simulink model "SoRo_Compliant_Demo_0906"  (R2023b)
settings: Solver=FixedStepAuto  StartTime=0.0  StopTime=inf  FixedStep=0.01  RelTol=1e-3
undefined symbols (not defined in the file): Down, Pull
libraries: simulink x50, speedgoatlib_IO691 x20, canmsglib x19, slpidlib x12, dspfdesign x6
(part 3 of 3)

== system SoRo_Compliant_Demo_0906/Tension_Mode_flag=2/Subsystem2 ==
  tension_in : Inport
  position_in : Inport  Port=2
  Enable : EnablePort
  tension_out : Outport
  position_out : Outport  Port=2
  wires:
  position_in/1 -> position_out/1
  tension_in/1 -> tension_out/1

== system SoRo_Compliant_Demo_0906/Tension_Mode_flag=2/Subsystem3 ==
  tension_in : Inport
  position_in : Inport  Port=2
  Enable : EnablePort
  tension_out : Outport
  position_out : Outport  Port=2
  wires:
  tension_in/1 -> tension_out/1
  position_in/1 -> position_out/1

== system SoRo_Compliant_Demo_0906/Tension_adjust_flag=4/Subsystem1 ==
  InitialSwitchValue_in : Inport
  Enable : EnablePort
  InitialSwitchValue_out : Outport
  wires:
  InitialSwitchValue_in/1 -> InitialSwitchValue_out/1

== system SoRo_Compliant_Demo_0906/Tension_adjust_flag=4/Subsystem4 ==
  tension_in : Inport
  position_in : Inport  Port=2
  Enable : EnablePort
  tension_out : Outport
  position_out : Outport  Port=2
  wires:
  tension_in/1 -> tension_out/1
  position_in/1 -> position_out/1

== system SoRo_Compliant_Demo_0906/Tension_adjust_flag=4/Subsystem5 ==
  tension_in : Inport
  position_in : Inport  Port=2
  Enable : EnablePort
  tension_out : Outport
  position_out : Outport  Port=2
  wires:
  tension_in/1 -> tension_out/1
  position_in/1 -> position_out/1

== system SoRo_Compliant_Demo_0906/Tension_adjust_flag=4/Subsystem6 ==
  tension_in : Inport
  position_in : Inport  Port=2
  Enable : EnablePort
  tension_out : Outport
  position_out : Outport  Port=2
  wires:
  position_in/1 -> position_out/1
  tension_in/1 -> tension_out/1

== system SoRo_Compliant_Demo_0906/Tension_adjust_flag=4/Subsystem7 ==
  tension_in : Inport
  position_in : Inport  Port=2
  Enable : EnablePort
  tension_out : Outport
  position_out : Outport  Port=2
  wires:
  tension_in/1 -> tension_out/1
  position_in/1 -> position_out/1

== system SoRo_Compliant_Demo_0906/Transmit/Driver_Upload ==
  Enable : EnablePort  StatesWhenEnabling=reset
  CAN Pack : canmsglib/CAN Pack  CANdbFile=E:\OneDrive\OneDrive - The Chinese University of Hong Kong\文档\Research\SRIL\12nd\Experiment\Simulink\RoboModule0729.dbc  MsgList=Configuration_all  MsgName=Configuration_all  MsgIDType=Standard (11-bit identifier)  MsgIdentifier=10  MsgLength=8  Remote=off  ApplyMinMax=off  BusOutput=off  SignalInfo={'Data2','16','8','BE','unsigned','Standard','0','1','0','-Inf','Inf';'Data3','24','8','BE','unsigned','Standard','0','1','0','-Inf','Inf';'Data4','32','8','BE','unsigned','Standard','0','1','0','-Inf','Inf';'Data5','40','8','BE','unsigned','Standard','0','1','0','-Inf','Inf';'Data6','48','8','BE','unsigned','Standard','0','1','0','-Inf','Inf';'Data7','56','8','BE','unsigned','Standard','0','1','0','-Inf','Inf';'output_cycle_curvelpos','0','8','BE','unsigned','Standard','0','1','0','-Inf','Inf';'output_cycle_others','8','8','BE','unsigned','Standard','0','1','0','-Inf','Inf'}
      settings: DataFormat=CANdb specified signals
  "CAN Write " : speedgoatlib_IO691/CAN Write   moduleType=IO691  id=1  channel=1  canType=CAN (HS)  messageType=CAN (HS)  useBusIn=off  numOfMsg=1  enableInput=off  enableStatusPort=off  ts=-1  initValues=[691 1 -1 0 1 1 0 1 0 0]
      settings: SourceProductName=Simulink Real-Time: Speedgoat I/O Blockset
  Constant4 : Constant  Value=hex2dec('0x55')  OutDataTypeStr=uint8  SampleTime=-1
  Constant5 : Constant  Value=hex2dec('0x64')  OutDataTypeStr=uint8  SampleTime=-1
  Constant6 : Constant  Value=hex2dec('0x00')  OutDataTypeStr=uint8  SampleTime=-1
  wires:
  CAN Pack/1 -> "CAN Write "/1
  Constant4/1 -> CAN Pack/1, CAN Pack/3, CAN Pack/5, CAN Pack/6, CAN Pack/4, CAN Pack/2
  Constant5/1 -> CAN Pack/7
  Constant6/1 -> CAN Pack/8

== system SoRo_Compliant_Demo_0906/Transmit/Mode Selection ==
  Enable : EnablePort  StatesWhenEnabling=reset
  CAN Pack : canmsglib/CAN Pack  CANdbFile=E:\Research\SRIL\12nd\Simulink\RoboModule0729.dbc  MsgList=Mode_Selection_all  MsgName=Mode_Selection_all  MsgIDType=Standard (11-bit identifier)  MsgIdentifier=1  MsgLength=8  Remote=off  ApplyMinMax=off  BusOutput=off  SignalInfo={'Data1','8','8','BE','unsigned','Standard','0','1','0','-Inf','Inf';'Data2','16','8','BE','unsigned','Standard','0','1','0','-Inf','Inf';'Data3','24','8','BE','unsigned','Standard','0','1','0','-Inf','Inf';'Data4','32','8','BE','unsigned','Standard','0','1','0','-Inf','Inf';'Data5','40','8','BE','unsigned','Standard','0','1','0','-Inf','Inf';'Data6','48','8','BE','unsigned','Standard','0','1','0','-Inf','Inf';'Data7','56','8','BE','unsigned','Standard','0','1','0','-Inf','Inf';'Mode','0','8','BE','unsigned','Standard','0','1','0','-Inf','Inf'}
      settings: DataFormat=CANdb specified signals
  "CAN Write " : speedgoatlib_IO691/CAN Write   moduleType=IO691  id=1  channel=1  canType=CAN (HS)  messageType=CAN (HS)  useBusIn=off  numOfMsg=1  enableInput=off  enableStatusPort=off  ts=-1  initValues=[691 1 -1 0 1 1 0 1 0 0]
      settings: SourceProductName=Simulink Real-Time: Speedgoat I/O Blockset
  Constant2 : Constant  Value=hex2dec('0x55')  OutDataTypeStr=uint8  SampleTime=-1
  Mode Number1 : Constant  Value=hex2dec('0x04')  OutDataTypeStr=uint8  SampleTime=-1
  wires:
  Constant2/1 -> CAN Pack/1, CAN Pack/3, CAN Pack/5, CAN Pack/6, CAN Pack/7, CAN Pack/4, CAN Pack/2
  CAN Pack/1 -> "CAN Write "/1
  Mode Number1/1 -> CAN Pack/8

== system SoRo_Compliant_Demo_0906/Transmit/PosSpdMode1 ==
  note: R ated Voltage of Motor is 12 V. Supply Voltage is 24 V. Limilation of the temp_pwm is set as 2500.
  Inport2 : Inport
  Enable : EnablePort
  CAN Pack : canmsglib/CAN Pack  CANdbFile=E:\OneDrive\OneDrive - The Chinese University of Hong Kong\文档\Research\SRIL\12nd\Experiment\Simulink\RoboModule0729.dbc  MsgList=Position_Dr1  MsgName=Position_Dr1  MsgIDType=Standard (11-bit identifier)  MsgIdentifier=21  MsgLength=8  Remote=off  ApplyMinMax=off  BusOutput=off  SignalInfo={'Data2','16','8','BE','unsigned','Standard','0','1','0','-Inf','Inf';'Data3','24','8','BE','unsigned','Standard','0','1','0','-Inf','Inf';'temp_position','56','32','BE','signed','Standard','0','1','0','-Inf','Inf';'temp_pwm','8','16','BE','unsigned','Standard','0','1','0','-Inf','Inf'}
      settings: DataFormat=CANdb specified signals
  "CAN Write " : speedgoatlib_IO691/CAN Write   moduleType=IO691  id=1  channel=1  canType=CAN (HS)  messageType=CAN (HS)  useBusIn=off  numOfMsg=1  enableInput=off  enableStatusPort=off  ts=-1  initValues=[691 1 -1 0 1 1 0 1 0 0]
      settings: SourceProductName=Simulink Real-Time: Speedgoat I/O Blockset
  Constant1 : Constant  Value=5000
  Constant3 : Constant  Value=hex2dec('0x55')  OutDataTypeStr=uint8  SampleTime=-1
  wires:
  Constant3/1 -> CAN Pack/2, CAN Pack/1
  Inport2/1 -> CAN Pack/3
  Constant1/1 -> CAN Pack/4
  CAN Pack/1 -> "CAN Write "/1

== system SoRo_Compliant_Demo_0906/Transmit/PosSpdMode2 ==
  note: R ated Voltage of Motor is 12 V. Supply Voltage is 24 V. Limilation of the temp_pwm is set as 2500.
  Inport2 : Inport
  Enable : EnablePort
  CAN Pack : canmsglib/CAN Pack  CANdbFile=E:\Research\SRIL\12nd\Simulink\RoboModule0729.dbc  MsgList=Position_Dr2  MsgName=Position_Dr2  MsgIDType=Standard (11-bit identifier)  MsgIdentifier=37  MsgLength=8  Remote=off  ApplyMinMax=off  BusOutput=off  SignalInfo={'Data2','16','8','BE','unsigned','Standard','0','1','0','-Inf','Inf';'Data3','24','8','BE','unsigned','Standard','0','1','0','-Inf','Inf';'temp_position','56','32','BE','signed','Standard','0','1','0','-Inf','Inf';'temp_pwm','8','16','BE','unsigned','Standard','0','1','0','-Inf','Inf'}
      settings: DataFormat=CANdb specified signals
  "CAN Write " : speedgoatlib_IO691/CAN Write   moduleType=IO691  id=1  channel=1  canType=CAN (HS)  messageType=CAN (HS)  useBusIn=off  numOfMsg=1  enableInput=off  enableStatusPort=off  ts=-1  initValues=[691 1 -1 0 1 1 0 1 0 0]
      settings: SourceProductName=Simulink Real-Time: Speedgoat I/O Blockset
  Constant1 : Constant  Value=5000
  Constant3 : Constant  Value=hex2dec('0x55')  OutDataTypeStr=uint8  SampleTime=-1
  Scope : Scope
  wires:
  CAN Pack/1 -> "CAN Write "/1
  Constant3/1 -> CAN Pack/2, CAN Pack/1
  Inport2/1 -> Scope/1, CAN Pack/3
  Constant1/1 -> CAN Pack/4

== system SoRo_Compliant_Demo_0906/Transmit/PosSpdMode3 ==
  note: R ated Voltage of Motor is 12 V. Supply Voltage is 24 V. Limilation of the temp_pwm is set as 2500.
  Inport2 : Inport
  Enable : EnablePort
  CAN Pack : canmsglib/CAN Pack  CANdbFile=E:\OneDrive\OneDrive - The Chinese University of Hong Kong\文档\Research\SRIL\12nd\Experiment\Simulink\RoboModule0729.dbc  MsgList=Position_Dr3  MsgName=Position_Dr3  MsgIDType=Standard (11-bit identifier)  MsgIdentifier=53  MsgLength=8  Remote=off  ApplyMinMax=off  BusOutput=off  SignalInfo={'Data2','16','8','BE','unsigned','Standard','0','1','0','-Inf','Inf';'Data3','24','8','BE','unsigned','Standard','0','1','0','-Inf','Inf';'temp_position','56','32','BE','signed','Standard','0','1','0','-Inf','Inf';'temp_pwm','8','16','BE','unsigned','Standard','0','1','0','-Inf','Inf'}
      settings: DataFormat=CANdb specified signals
  "CAN Write " : speedgoatlib_IO691/CAN Write   moduleType=IO691  id=1  channel=1  canType=CAN (HS)  messageType=CAN (HS)  useBusIn=off  numOfMsg=1  enableInput=off  enableStatusPort=off  ts=-1  initValues=[691 1 -1 0 1 1 0 1 0 0]
      settings: SourceProductName=Simulink Real-Time: Speedgoat I/O Blockset
  Constant1 : Constant  Value=5000
  Constant3 : Constant  Value=hex2dec('0x55')  OutDataTypeStr=uint8  SampleTime=-1
  wires:
  CAN Pack/1 -> "CAN Write "/1
  Constant3/1 -> CAN Pack/2, CAN Pack/1
  Inport2/1 -> CAN Pack/3
  Constant1/1 -> CAN Pack/4

== system SoRo_Compliant_Demo_0906/Transmit/PosSpdMode4 ==
  note: R ated Voltage of Motor is 12 V. Supply Voltage is 24 V. Limilation of the temp_pwm is set as 2500.
  Inport2 : Inport
  Enable : EnablePort
  CAN Pack : canmsglib/CAN Pack  CANdbFile=E:\OneDrive\OneDrive - The Chinese University of Hong Kong\文档\Research\SRIL\12nd\Experiment\Simulink\RoboModule0729.dbc  MsgList=Position_Dr4  MsgName=Position_Dr4  MsgIDType=Standard (11-bit identifier)  MsgIdentifier=69  MsgLength=8  Remote=off  ApplyMinMax=off  BusOutput=off  SignalInfo={'Data2','16','8','BE','unsigned','Standard','0','1','0','-Inf','Inf';'Data3','24','8','BE','unsigned','Standard','0','1','0','-Inf','Inf';'temp_position','56','32','BE','signed','Standard','0','1','0','-Inf','Inf';'temp_pwm','8','16','BE','unsigned','Standard','0','1','0','-Inf','Inf'}
      settings: DataFormat=CANdb specified signals
  "CAN Write " : speedgoatlib_IO691/CAN Write   moduleType=IO691  id=1  channel=1  canType=CAN (HS)  messageType=CAN (HS)  useBusIn=off  numOfMsg=1  enableInput=off  enableStatusPort=off  ts=-1  initValues=[691 1 -1 0 1 1 0 1 0 0]
      settings: SourceProductName=Simulink Real-Time: Speedgoat I/O Blockset
  Constant1 : Constant  Value=5000
  Constant3 : Constant  Value=hex2dec('0x55')  OutDataTypeStr=uint8  SampleTime=-1
  wires:
  CAN Pack/1 -> "CAN Write "/1
  Constant3/1 -> CAN Pack/2, CAN Pack/1
  Inport2/1 -> CAN Pack/3
  Constant1/1 -> CAN Pack/4

== system SoRo_Compliant_Demo_0906/Transmit/PosSpdMode5 ==
  note: R ated Voltage of Motor is 12 V. Supply Voltage is 24 V. Limilation of the temp_pwm is set as 2500.
  Inport2 : Inport
  Enable : EnablePort
  CAN Pack : canmsglib/CAN Pack  CANdbFile=E:\OneDrive\OneDrive - The Chinese University of Hong Kong\文档\Research\SRIL\12nd\Experiment\Simulink\RoboModule0729.dbc  MsgList=Position_Dr5  MsgName=Position_Dr5  MsgIDType=Standard (11-bit identifier)  MsgIdentifier=85  MsgLength=8  Remote=off  ApplyMinMax=off  BusOutput=off  SignalInfo={'Data2','16','8','BE','unsigned','Standard','0','1','0','-Inf','Inf';'Data3','24','8','BE','unsigned','Standard','0','1','0','-Inf','Inf';'temp_position','56','32','BE','signed','Standard','0','1','0','-Inf','Inf';'temp_pwm','8','16','BE','unsigned','Standard','0','1','0','-Inf','Inf'}
      settings: DataFormat=CANdb specified signals
  "CAN Write " : speedgoatlib_IO691/CAN Write   moduleType=IO691  id=1  channel=1  canType=CAN (HS)  messageType=CAN (HS)  useBusIn=off  numOfMsg=1  enableInput=off  enableStatusPort=off  ts=-1  initValues=[691 1 -1 0 1 1 0 1 0 0]
      settings: SourceProductName=Simulink Real-Time: Speedgoat I/O Blockset
  Constant1 : Constant  Value=5000
  Constant3 : Constant  Value=hex2dec('0x55')  OutDataTypeStr=uint8  SampleTime=-1
  Scope : Scope
  wires:
  CAN Pack/1 -> "CAN Write "/1
  Constant3/1 -> CAN Pack/2, CAN Pack/1
  Inport2/1 -> Scope/1, CAN Pack/3
  Constant1/1 -> CAN Pack/4

== system SoRo_Compliant_Demo_0906/Transmit/Reset ==
  Enable : EnablePort  StatesWhenEnabling=reset
  CAN Pack : canmsglib/CAN Pack  CANdbFile=E:\Research\SRIL\12nd\Simulink\RoboModule0729.dbc  MsgList=Reset_all  MsgName=Reset_all  MsgIDType=Standard (11-bit identifier)  MsgIdentifier=0  MsgLength=8  Remote=off  ApplyMinMax=off  BusOutput=off  SignalInfo={'Data0','0','8','BE','unsigned','Standard','0','1','0','-Inf','Inf';'Data1','8','8','BE','unsigned','Standard','0','1','0','-Inf','Inf';'Data2','16','8','BE','unsigned','Standard','0','1','0','-Inf','Inf';'Data3','24','8','BE','unsigned','Standard','0','1','0','-Inf','Inf';'Data4','32','8','BE','unsigned','Standard','0','1','0','-Inf','Inf';'Data5','40','8','BE','unsigned','Standard','0','1','0','-Inf','Inf';'Data6','48','8','BE','unsigned','Standard','0','1','0','-Inf','Inf';'Data7','56','8','BE','unsigned','Standard','0','1','0','-Inf','Inf'}
      settings: DataFormat=CANdb specified signals
  "CAN Write " : speedgoatlib_IO691/CAN Write   moduleType=IO691  id=1  channel=1  canType=CAN (HS)  messageType=CAN (HS)  useBusIn=off  numOfMsg=1  enableInput=off  enableStatusPort=off  ts=-1  initValues=[691 1 -1 0 1 1 0 1 0 0]
      settings: SourceProductName=Simulink Real-Time: Speedgoat I/O Blockset
  Constant2 : Constant  Value=hex2dec('0x55')  OutDataTypeStr=uint8  SampleTime=-1
  wires:
  CAN Pack/1 -> "CAN Write "/1
  Constant2/1 -> CAN Pack/1, CAN Pack/3, CAN Pack/5, CAN Pack/6, CAN Pack/7, CAN Pack/8, CAN Pack/4, CAN Pack/2

== system SoRo_Compliant_Demo_0906/Transmit/Reset_Manually ==
  Enable : EnablePort  StatesWhenEnabling=reset
  Trigger : TriggerPort  VariantControl=(inherit)  PortDimensions=1
  CAN Pack : canmsglib/CAN Pack  CANdbFile=E:\OneDrive\OneDrive - The Chinese University of Hong Kong\文档\Research\SRIL\12nd\Experiment\Simulink\RoboModule0729.dbc  MsgList=Reset_all  MsgName=Reset_all  MsgIDType=Standard (11-bit identifier)  MsgIdentifier=0  MsgLength=8  Remote=off  ApplyMinMax=off  BusOutput=off  SignalInfo={'Data0','0','8','BE','unsigned','Standard','0','1','0','-Inf','Inf';'Data1','8','8','BE','unsigned','Standard','0','1','0','-Inf','Inf';'Data2','16','8','BE','unsigned','Standard','0','1','0','-Inf','Inf';'Data3','24','8','BE','unsigned','Standard','0','1','0','-Inf','Inf';'Data4','32','8','BE','unsigned','Standard','0','1','0','-Inf','Inf';'Data5','40','8','BE','unsigned','Standard','0','1','0','-Inf','Inf';'Data6','48','8','BE','unsigned','Standard','0','1','0','-Inf','Inf';'Data7','56','8','BE','unsigned','Standard','0','1','0','-Inf','Inf'}
      settings: DataFormat=CANdb specified signals
  "CAN Write " : speedgoatlib_IO691/CAN Write   moduleType=IO691  id=1  channel=1  canType=CAN (HS)  messageType=CAN (HS)  useBusIn=off  numOfMsg=1  enableInput=off  enableStatusPort=off  ts=-1  initValues=[691 1 -1 0 1 1 0 1 0 0]
      settings: SourceProductName=Simulink Real-Time: Speedgoat I/O Blockset
  Constant2 : Constant  Value=hex2dec('0x55')  OutDataTypeStr=uint8  SampleTime=-1
  wires:
  CAN Pack/1 -> "CAN Write "/1
  Constant2/1 -> CAN Pack/1, CAN Pack/3, CAN Pack/5, CAN Pack/6, CAN Pack/7, CAN Pack/8, CAN Pack/4, CAN Pack/2

== system SoRo_Compliant_Demo_0906/Displacement_mode_flag=5/Displacement_mode_flag=0/Subsystem1 ==
  position_in : Inport
  Enable : EnablePort
  position_out : Outport
  wires:
  position_in/1 -> position_out/1

== system SoRo_Compliant_Demo_0906/Displacement_mode_flag=5/Displacement_mode_flag=0/Subsystem2 ==
  position_in : Inport
  Enable : EnablePort
  position_out : Outport
  wires:
  position_in/1 -> position_out/1

== system SoRo_Compliant_Demo_0906/Displacement_mode_flag=5/Displacement_mode_flag=0/Subsystem3 ==
  position_in : Inport
  Enable : EnablePort
  position_out : Outport
  wires:
  position_in/1 -> position_out/1

== system SoRo_Compliant_Demo_0906/Displacement_mode_flag=5/Displacement_mode_flag=0/Subsystem5 ==
  position_in : Inport
  Enable : EnablePort
  position_out : Outport
  wires:
  position_in/1 -> position_out/1

== system SoRo_Compliant_Demo_0906/Displacement_mode_flag=5/Displacement_mode_flag=1/Subsystem1 ==
  position_in : Inport
  Enable : EnablePort
  position_out : Outport
  wires:
  position_in/1 -> position_out/1

== system SoRo_Compliant_Demo_0906/Displacement_mode_flag=5/Displacement_mode_flag=1/Subsystem2 ==
  position_in : Inport
  Enable : EnablePort
  position_out : Outport
  wires:
  position_in/1 -> position_out/1

== system SoRo_Compliant_Demo_0906/Displacement_mode_flag=5/Displacement_mode_flag=1/Subsystem3 ==
  position_in : Inport
  Enable : EnablePort
  position_out : Outport
  wires:
  position_in/1 -> position_out/1

== system SoRo_Compliant_Demo_0906/Displacement_mode_flag=5/Displacement_mode_flag=1/Subsystem5 ==
  position_in : Inport
  Enable : EnablePort
  position_out : Outport
  wires:
  position_in/1 -> position_out/1

== system SoRo_Compliant_Demo_0906/Displacement_mode_flag=5/Displacement_mode_flag=2/Subsystem1 ==
  position_in : Inport
  Enable : EnablePort
  position_out : Outport
  wires:
  position_in/1 -> position_out/1

== system SoRo_Compliant_Demo_0906/Displacement_mode_flag=5/Displacement_mode_flag=2/Subsystem2 ==
  position_in : Inport
  Enable : EnablePort
  position_out : Outport
  wires:
  position_in/1 -> position_out/1

== system SoRo_Compliant_Demo_0906/Displacement_mode_flag=5/Displacement_mode_flag=2/Subsystem3 ==
  position_in : Inport
  Enable : EnablePort
  position_out : Outport
  wires:
  position_in/1 -> position_out/1

== system SoRo_Compliant_Demo_0906/Displacement_mode_flag=5/Displacement_mode_flag=2/Subsystem5 ==
  position_in : Inport
  Enable : EnablePort
  position_out : Outport
  wires:
  position_in/1 -> position_out/1

== system SoRo_Compliant_Demo_0906/Displacement_mode_flag=5/Displacement_mode_flag=3/Subsystem1 ==
  position_in : Inport
  Enable : EnablePort
  position_out : Outport
  wires:
  position_in/1 -> position_out/1

== system SoRo_Compliant_Demo_0906/Displacement_mode_flag=5/Displacement_mode_flag=3/Subsystem2 ==
  position_in : Inport
  Enable : EnablePort
  position_out : Outport
  wires:
  position_in/1 -> position_out/1

== system SoRo_Compliant_Demo_0906/Displacement_mode_flag=5/Displacement_mode_flag=3/Subsystem3 ==
  position_in : Inport
  Enable : EnablePort
  position_out : Outport
  wires:
  position_in/1 -> position_out/1

== system SoRo_Compliant_Demo_0906/Displacement_mode_flag=5/Displacement_mode_flag=3/Subsystem5 ==
  position_in : Inport
  Enable : EnablePort
  position_out : Outport
  wires:
  position_in/1 -> position_out/1

== system SoRo_Compliant_Demo_0906/Displacement_mode_flag=5/Displacement_mode_flag=4/Subsystem1 ==
  position_in : Inport
  Enable : EnablePort
  position_out : Outport
  wires:
  position_in/1 -> position_out/1

== system SoRo_Compliant_Demo_0906/Displacement_mode_flag=5/Displacement_mode_flag=4/Subsystem2 ==
  position_in : Inport
  Enable : EnablePort
  position_out : Outport
  wires:
  position_in/1 -> position_out/1

== system SoRo_Compliant_Demo_0906/Displacement_mode_flag=5/Displacement_mode_flag=4/Subsystem3 ==
  position_in : Inport
  Enable : EnablePort
  position_out : Outport
  wires:
  position_in/1 -> position_out/1

== system SoRo_Compliant_Demo_0906/Displacement_mode_flag=5/Displacement_mode_flag=4/Subsystem5 ==
  position_in : Inport
  Enable : EnablePort
  position_out : Outport
  wires:
  position_in/1 -> position_out/1

== stateflow chart SoRo_Compliant_Demo_0906/Chart2 ==
  settings: sampleTime=0.001
  note: Operation logic: The initial flag is 0. Imitating the operation logic of the drone, long press the H switch for 5 seconds, the flag changes to 1, and the system starts. Long press again for 5 seconds, and the flag changes back to 0.
  state b [parallel]
    settings: executionOrder=1
    state off
      during:flag=0;
    state Initial
      during:flag=1;
    state Tension_Mode
      during:flag=2;
    state Displacement_Mode
      during:flag=3;
    state Individual_Adjust
      during:flag=5;
    state Stiffness_Adjust
      during:flag=4;
    state Emergency_Brake
      during:flag=6;
    Individual_Adjust -> off [order 3] : [duration(Switch_H > 1000) > 3]
    Displacement_Mode -> off [order 2] : [duration(Switch_H > 1000) > 3]
    Tension_Mode -> off [order 3] : [duration(Switch_H > 1000) > 3]
    Displacement_Mode -> Tension_Mode [order 1] : [Switch_B_Change > 0]
    Displacement_Mode -> Individual_Adjust [order 4] : [Switch_D_Change > 0]
    Initial -> Tension_Mode [order 2] : [Switch_A_Change > 0]
    Initial -> off [order 1] : [duration(Switch_H > 1000) > 3]
    (default) -> off
    Tension_Mode -> Initial [order 1] : [Switch_A_Change > 0]
    Individual_Adjust -> Displacement_Mode [order 1] : [Switch_D_Change > 0]
    off -> Initial : [duration(Switch_H > 1000) > 3]
    Tension_Mode -> Displacement_Mode [order 2] : [Switch_B_Change > 0]
    Initial -> Emergency_Brake [order 3] : [Switch_C_Change > 0]
    Tension_Mode -> Stiffness_Adjust [order 5] : [Switch_E_Change > 0]
    Stiffness_Adjust -> Tension_Mode [order 3] : [Switch_E_Change > 0]
    Tension_Mode -> Emergency_Brake [order 4] : [Switch_C_Change > 0]
    Displacement_Mode -> Emergency_Brake [order 3] : [Switch_C_Change > 0]
    Individual_Adjust -> Emergency_Brake [order 2] : [Switch_C_Change > 0]
    Stiffness_Adjust -> off [order 1] : [duration(Switch_H > 1000) > 3]
    Stiffness_Adjust -> Emergency_Brake [order 2] : [Switch_C_Change > 0]
  data: flag output double; Switch_A_Change input double; Switch_E_Change input double; Switch_H input double; Switch_B_Change input double; Switch_C_Change input double; Switch_D_Change input double

== matlab function SoRo_Compliant_Demo_0906/MATLAB Function4 ==
  data: y output; u_out output; u input; u_last input
function [y,u_out] = fcn(u,u_last)
if abs(u-u_last)>20
    y = 1;
else
    y = 0;
end
u_out = u;

== matlab function SoRo_Compliant_Demo_0906/Tension_Mode_flag=2/MATLAB Function1 ==
  data: y output; u input; threshold input
function y = noise_reduction(u,threshold)
if abs(u - 1000) > threshold
    y = u;
else
    y = 1000;
end

== matlab function SoRo_Compliant_Demo_0906/MATLAB Function1 ==
  data: y output; u_out output; u input; u_last input
function [y,u_out] = fcn(u,u_last)
if abs(u-u_last)>20
    y = 1;
else
    y = 0;
end
u_out = u;

== matlab function SoRo_Compliant_Demo_0906/MATLAB Function2 ==
  data: y output; u_out output; u input; u_last input
function [y,u_out] = fcn(u,u_last)
if abs(u-u_last)>20
    y = 1;
else
    y = 0;
end
u_out = u;

== matlab function SoRo_Compliant_Demo_0906/MATLAB Function3 ==
  data: y output; u_out output; u input; u_last input
function [y,u_out] = fcn(u,u_last)
if abs(u-u_last)>20
    y = 1;
else
    y = 0;
end
u_out = u;

== matlab function SoRo_Compliant_Demo_0906/Tension_Mode_flag=2/MATLAB Function2 ==
  data: y output; u input; threshold input
function y = noise_reduction(u,threshold)
if abs(u - 1000) > threshold
    y = u;
else
    y = 1000;
end

== matlab function SoRo_Compliant_Demo_0906/Tension_adjust_flag=4/MATLAB Function1 ==
  data: otpt_last input; y output; u input; threshold input; initial input
function y = noise_reduction(otpt_last,u,threshold,initial)
if abs(u - initial) > threshold
    if abs(u - otpt_last) > threshold
        y = u;
    else
        y = otpt_last;
    end
else
    y = initial;
end

== matlab function SoRo_Compliant_Demo_0906/Displacement_mode_flag=3/MATLAB Function1 ==
  data: y output; u input; threshold input
function y = noise_reduction(u,threshold)
if abs(u - 1000) > threshold
    y = u;
else
    y = 1000;
end

== matlab function SoRo_Compliant_Demo_0906/Displacement_mode_flag=3/MATLAB Function2 ==
  data: y output; u input; threshold input
function y = noise_reduction(u,threshold)
if abs(u - 1000) > threshold
    y = u;
else
    y = 1000;
end

== matlab function SoRo_Compliant_Demo_0906/Subsystem/MATLAB Function5 ==
  data: y output; u input; threshold input
function y = noise_reduction(u,threshold)
if abs(u - 1000) > threshold
    y = u;
else
    y = 1000;
end

== matlab function SoRo_Compliant_Demo_0906/MATLAB Function6 ==
  data: y output; u_out output; u input; u_last input
function [y,u_out] = fcn(u,u_last)
if abs(u-u_last)>20
    y = 1;
else
    y = 0;
end
u_out = u;

== matlab function SoRo_Compliant_Demo_0906/Displacement_mode_flag=5/Displacement_mode_flag=1/MATLAB Function1 ==
  data: y output; u input; threshold input
function y = noise_reduction(u,threshold)
if abs(u - 1000) > threshold
    y = u;
else
    y = 1000;
end

== matlab function SoRo_Compliant_Demo_0906/Displacement_mode_flag=5/Displacement_mode_flag=2/MATLAB Function1 ==
  data: y output; u input; threshold input
function y = noise_reduction(u,threshold)
if abs(u - 1000) > threshold
    y = u;
else
    y = 1000;
end

== stateflow chart SoRo_Compliant_Demo_0906/Displacement_mode_flag=5/Chart2 ==
  settings: sampleTime=0.001
  state b [parallel]
    settings: executionOrder=1
    state LeftMotor4
      during:flag_direction=4;
    state RightMotor1
      during:flag_direction=1;
    state off
      during:flag_direction=0;
    state UpMotor3
      during:flag_direction=3;
    state DownMotor2
      during:flag_direction=2;
    LeftMotor4 -> off : [duration(LeftMotor4_RightMotor1 < 400) > 1|| reset > 0]
    off -> LeftMotor4 [order 1] : [duration(LeftMotor4_RightMotor1 < 400) > 1]
    RightMotor1 -> off : [duration(LeftMotor4_RightMotor1 > 1600) > 1 || reset > 0]
    (default) -> off
    off -> RightMotor1 [order 2] : [duration(LeftMotor4_RightMotor1 > 1600) > 1]
    off -> DownMotor2 [order 4] : [duration(UpMotor3_DownMotor2 > 1600) > 1]
    DownMotor2 -> off : [duration(UpMotor3_DownMotor2 > 1600) > 1 || reset > 0]
    off -> UpMotor3 [order 3] : [duration(UpMotor3_DownMotor2 < 400) > 1]
    UpMotor3 -> off : [duration(UpMotor3_DownMotor2 < 400) > 1 || reset > 0]
  data: flag_direction output double; LeftMotor4_RightMotor1 input double; UpMotor3_DownMotor2 input double; reset input boolean

== matlab function SoRo_Compliant_Demo_0906/Displacement_mode_flag=5/Displacement_mode_flag=3/MATLAB Function1 ==
  data: y output; u input; threshold input
function y = noise_reduction(u,threshold)
if abs(u - 1000) > threshold
    y = u;
else
    y = 1000;
end

== matlab function SoRo_Compliant_Demo_0906/Displacement_mode_flag=5/Displacement_mode_flag=4/MATLAB Function1 ==
  data: y output; u input; threshold input
function y = noise_reduction(u,threshold)
if abs(u - 1000) > threshold
    y = u;
else
    y = 1000;
end

== matlab function SoRo_Compliant_Demo_0906/MATLAB Function7 ==
  data: y output; u input; u_last input
function y = fcn(u,u_last)
if abs(u-u_last)>200
    y = u_last;
else
    y = u;
end

== matlab function SoRo_Compliant_Demo_0906/MATLAB Function8 ==
  data: y output; u input; u_last input
function y = fcn(u,u_last)
if abs(u-u_last)>200
    y = u_last;
else
    y = u;
end

== matlab function SoRo_Compliant_Demo_0906/MATLAB Function9 ==
  data: y output; u input; u_last input
function y = fcn(u,u_last)
if abs(u-u_last)>200
    y = u_last;
else
    y = u;
end

== matlab function SoRo_Compliant_Demo_0906/MATLAB Function10 ==
  data: y output; u input; u_last input
function y = fcn(u,u_last)
if abs(u-u_last)>200
    y = u_last;
else
    y = u;
end

== matlab function SoRo_Compliant_Demo_0906/MATLAB Function11 ==
  data: y output; u input; u_last input
function y = fcn(u,u_last)
if abs(u-u_last)>200
    y = u_last;
else
    y = u;
end

== matlab function SoRo_Compliant_Demo_0906/Displacement_mode_flag=3/MATLAB Function3 ==
  data: y output; otpt_last input; reset input; inc input
function y = noise_reduction(otpt_last,reset,inc)
if reset > 0.5
    aa = 0;
else
    aa = otpt_last;
end
y = aa + inc;

== matlab function SoRo_Compliant_Demo_0906/MATLAB Function13 ==
  data: y output; u input; change input; u_last input
function y = fcn(u,change,u_last)
if change > 0
    y = u_last;
else
    y = u;
end

== matlab function SoRo_Compliant_Demo_0906/Displacement_mode_flag=3/MATLAB Function4 ==
  data: y output; otpt_last input; reset input; inc input
function y = noise_reduction(otpt_last,reset,inc)
if reset > 0.5
    aa = 0;
else
    aa = otpt_last;
end
y = aa + inc;

== matlab function SoRo_Compliant_Demo_0906/Displacement_mode_flag=5/Displacement_mode_flag=1/MATLAB Function4 ==
  data: y output; otpt_last input; reset input; inc input
function y = noise_reduction(otpt_last,reset,inc)
if reset > 0.5
    aa = 0;
else
    aa = otpt_last;
end
y = aa + inc;

== matlab function SoRo_Compliant_Demo_0906/Displacement_mode_flag=5/Displacement_mode_flag=2/MATLAB Function4 ==
  data: y output; otpt_last input; reset input; inc input
function y = noise_reduction(otpt_last,reset,inc)
if reset > 0.5
    aa = 0;
else
    aa = otpt_last;
end
y = aa + inc;

== matlab function SoRo_Compliant_Demo_0906/Displacement_mode_flag=5/Displacement_mode_flag=3/MATLAB Function4 ==
  data: y output; otpt_last input; reset input; inc input
function y = noise_reduction(otpt_last,reset,inc)
if reset > 0.5
    aa = 0;
else
    aa = otpt_last;
end
y = aa + inc;

== matlab function SoRo_Compliant_Demo_0906/Displacement_mode_flag=5/Displacement_mode_flag=4/MATLAB Function4 ==
  data: y output; otpt_last input; reset input; inc input
function y = noise_reduction(otpt_last,reset,inc)
if reset > 0.5
    aa = 0;
else
    aa = otpt_last;
end
y = aa + inc;

== matlab function SoRo_Compliant_Demo_0906/Tension_Mode_flag=2/MATLAB Function4 ==
  data: y output; otpt_last input; reset input; inc input
function y = noise_reduction(otpt_last,reset,inc)
if reset > 0.5
    aa = 0;
else
    aa = otpt_last;
end
y = aa + inc;

== matlab function SoRo_Compliant_Demo_0906/Tension_Mode_flag=2/MATLAB Function3 ==
  data: y output; otpt_last input; reset input; inc input
function y = noise_reduction(otpt_last,reset,inc)
if reset > 0.5
    aa = 0;
else
    aa = otpt_last;
end
y = aa + inc;

== matlab function SoRo_Compliant_Demo_0906/Subsystem/MATLAB Function4 ==
  data: y output; otpt_last input; inc input
function y = noise_reduction(otpt_last,inc)
    aa = otpt_last;
y = aa + inc;

== matlab function SoRo_Compliant_Demo_0906/Tension_Mode_flag=2/MATLAB Function5 ==
  data: y output; adj input; hold input; initial input
function y = saturation(adj,hold,initial)
if hold + adj < initial
    y = 0;
else
    y = adj;
end

== matlab function SoRo_Compliant_Demo_0906/Tension_Mode_flag=2/MATLAB Function6 ==
  data: y output; adj input; hold input; initial input
function y = saturation(adj,hold,initial)
if hold + adj < initial
    y = 0;
else
    y = adj;
end

== matlab function SoRo_Compliant_Demo_0906/Tension_Mode_flag=2/MATLAB Function7 ==
  data: y output; adj input; hold input; initial input
function y = saturation(adj,hold,initial)
if hold + adj < initial
    y = 0;
else
    y = adj;
end

== matlab function SoRo_Compliant_Demo_0906/Tension_Mode_flag=2/MATLAB Function8 ==
  data: y output; adj input; hold input; initial input
function y = saturation(adj,hold,initial)
if hold + adj < initial
    y = 0;
else
    y = adj;
end
